simulink library "posAng2RotMat_ul"  (R2022a)
settings: Solver=VariableStepAuto  StartTime=0.0  StopTime=10.0  RelTol=1e-3
libraries: sharedutil x2
settings Model: Creator=mcobb  LastModifiedBy=adabney
settings SolverCC: AlgebraicLoopSolver=TrustRegion
settings DebuggingCC: UnconnectedInputMsg=warning  UnconnectedOutputMsg=warning  UnconnectedLineMsg=warning  SFMachineParentedDataDiag=warning  ArithmeticOperatorsInVariantConditions=warning
settings SFSimCC: CustomCodeUndefinedFunction=UseInterfaceOnly

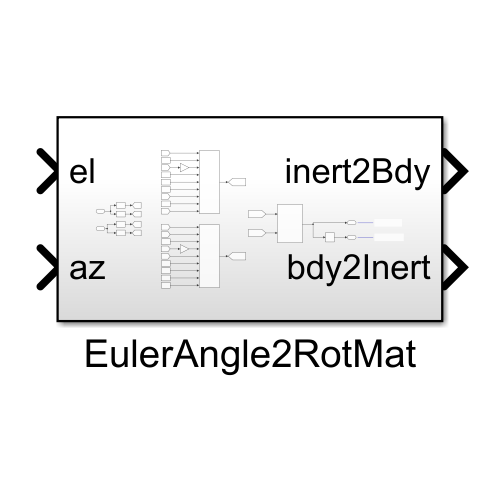
[thumbnail: Simulink's stored preview of the top-level diagram]
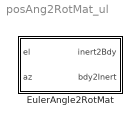
== system posAng2RotMat_ul ==
  EulerAngle2RotMat : Subsystem

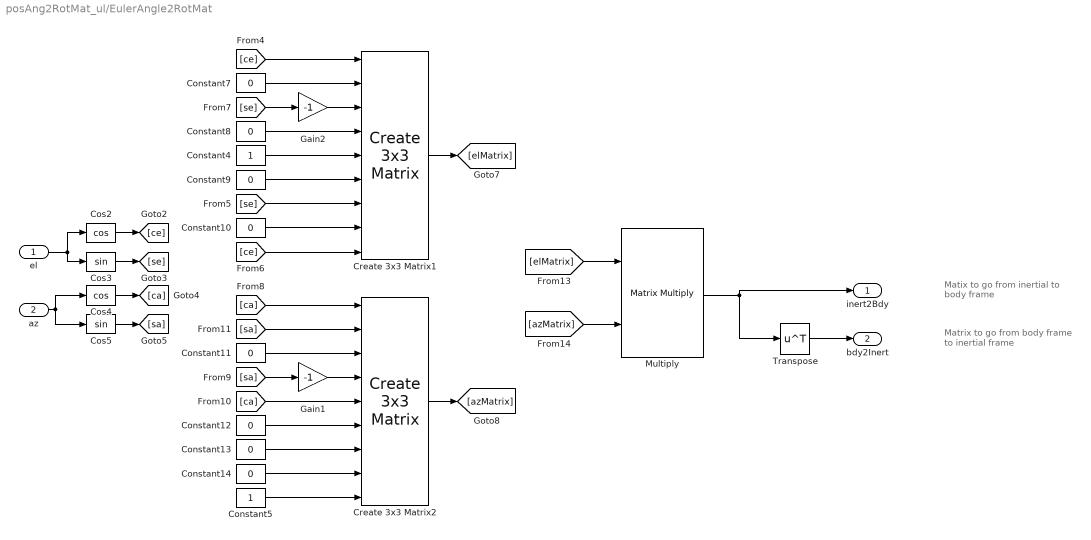
== system posAng2RotMat_ul/EulerAngle2RotMat ==
  note: Matrix to go from body
      | frame to inertial frame
  note: Matix to go from
      | inertial to body frame
  el : Inport
  az : Inport  Port=2
  Constant{7..14} (8 alike) : Constant  Value=0
  Constant4 : Constant
  Constant5 : Constant
  Cos2 : Trigonometry  Operator=cos
  Cos3 : Trigonometry
  Cos4 : Trigonometry  Operator=cos
  Cos5 : Trigonometry
  Create 3x3 Matrix1 : sharedutil/Create 3x3 Matrix  aMode=aMode
      settings: SourceProductBaseCode=AE,PW,DR,MT,VE
  Create 3x3 Matrix2 : sharedutil/Create 3x3 Matrix  aMode=aMode
      settings: SourceProductBaseCode=AE,PW,DR,MT,VE
  Gain1 : Gain  Gain=-1
  Gain2 : Gain  Gain=-1
  Multiply : Product  Multiplication=Matrix(*)
  Transpose : Math  Operator=transpose  SignedPower=on
  inert2Bdy : Outport  VectorParamsAs1DForOutWhenUnconnected=off
  bdy2Inert : Outport  Port=2  VectorParamsAs1DForOutWhenUnconnected=off
  wires:
  el/1 -> Cos3/1, Cos2/1
  az/1 -> Cos4/1, Cos5/1
  Cos2/1 -> [ce]
  Cos3/1 -> [se]
  Cos4/1 -> [ca]
  Cos5/1 -> [sa]
  Constant4/1 -> Create 3x3 Matrix1/5
  Constant5/1 -> Create 3x3 Matrix2/9
  Constant7/1 -> Create 3x3 Matrix1/2
  Constant8/1 -> Create 3x3 Matrix1/4
  Constant9/1 -> Create 3x3 Matrix1/6
  Constant10/1 -> Create 3x3 Matrix1/8
  Constant11/1 -> Create 3x3 Matrix2/3
  Constant12/1 -> Create 3x3 Matrix2/6
  Constant13/1 -> Create 3x3 Matrix2/7
  Constant14/1 -> Create 3x3 Matrix2/8
  [ce] -> Create 3x3 Matrix1/1
  [ce] -> Create 3x3 Matrix1/9
  [se] -> Gain2/1
  [se] -> Create 3x3 Matrix1/7
  [ca] -> Create 3x3 Matrix2/1
  [ca] -> Create 3x3 Matrix2/5
  [sa] -> Gain1/1
  Create 3x3 Matrix1/1 -> [elMatrix]
  Create 3x3 Matrix2/1 -> [azMatrix]
  Multiply/1 -> inert2Bdy/1, Transpose/1
  Transpose/1 -> bdy2Inert/1
  [elMatrix] -> Multiply/1
  [azMatrix] -> Multiply/2
  Gain1/1 -> Create 3x3 Matrix2/4
  [sa] -> Create 3x3 Matrix2/2
  Gain2/1 -> Create 3x3 Matrix1/3
